simulink model "masterAndSlaveRobots"  (R2021b)
settings: Solver=VariableStepAuto  StartTime=0.0  StopTime=5  RelTol=1e-3
undefined symbols (not defined in the file): A, Bm, Bs, Flp, Km, Ks, Mm, Ms
settings Model: Creator=riccardo  LastModifiedBy=riccardo

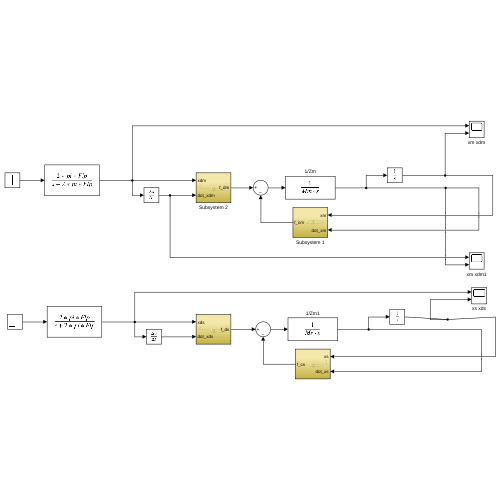
[thumbnail: Simulink's stored preview of the top-level diagram]
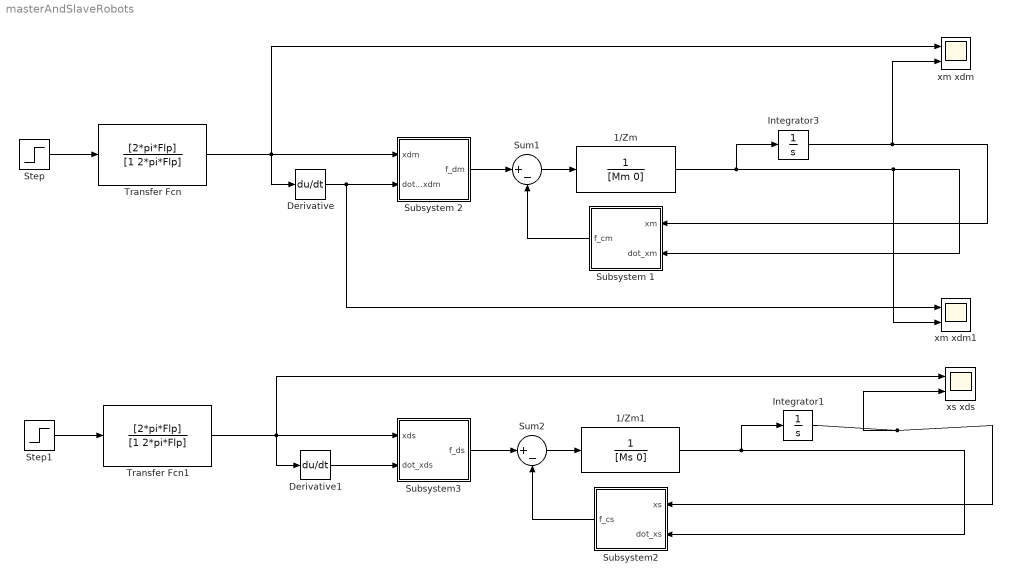
== system masterAndSlaveRobots ==
  1/Zm : TransferFcn  Denominator=[Mm 0]
  1/Zm1 : TransferFcn  Denominator=[Ms 0]
  Derivative : Derivative
  Derivative1 : Derivative
  Integrator1 : Integrator
  Integrator3 : Integrator
  Step : Step  Time=0.5  After=A  SampleTime=0
  Step1 : Step  Time=0.5  After=A  SampleTime=0
  Subsystem 1 : Subsystem
  Subsystem 2 : Subsystem
  Subsystem2 : Subsystem
  Subsystem3 : Subsystem
  Sum1 : Sum  Inputs=|+-
  Sum2 : Sum  Inputs=|+-
  Transfer Fcn : TransferFcn  Numerator=[2*pi*Flp]  Denominator=[1 2*pi*Flp]
  Transfer Fcn1 : TransferFcn  Numerator=[2*pi*Flp]  Denominator=[1 2*pi*Flp]
  xm xdm : Scope  NumInputPorts=2
  xm xdm1 : Scope  NumInputPorts=2
  xs xds : Scope  NumInputPorts=2
  wires:
  Sum1/1 -> 1/Zm/1
  1/Zm/1 -> xm xdm1/2, Subsystem 1/2(dot_xm), Integrator3/1
  Integrator3/1 -> xm xdm/2, Subsystem 1/1(xm)
  Subsystem 1/1(f_cm) -> Sum1/2
  Step/1 -> Transfer Fcn/1
  Transfer Fcn/1 -> xm xdm/1, Derivative/1, Subsystem 2/1(xdm)
  Derivative/1 -> xm xdm1/1, Subsystem 2/2(dot_xdm)
  Subsystem 2/1(f_dm) -> Sum1/1
  Subsystem2/1(f_cs) -> Sum2/2
  Sum2/1 -> 1/Zm1/1
  1/Zm1/1 -> Subsystem2/2(dot_xs), Integrator1/1
  Derivative1/1 -> Subsystem3/2(dot_xds)
  Integrator1/1 -> xs xds/2, Subsystem2/1(xs)
  Step1/1 -> Transfer Fcn1/1
  Subsystem3/1(f_ds) -> Sum2/1
  Transfer Fcn1/1 -> xs xds/1, Derivative1/1, Subsystem3/1(xds)

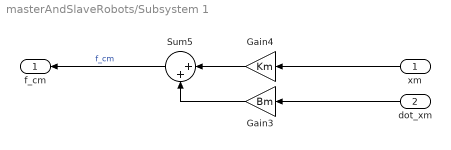
== system masterAndSlaveRobots/Subsystem 1 ==
  xm : Inport
  dot_xm : Inport  Port=2
  Gain3 : Gain  Gain=Bm
  Gain4 : Gain  Gain=Km
  Sum5 : Sum  Inputs=|++
  f_cm : Outport
  wires:
  Gain4/1 -> Sum5/1
  Gain3/1 -> Sum5/2
  dot_xm/1 -> Gain3/1
  Sum5/1 -> f_cm/1  "f_cm"
  xm/1 -> Gain4/1

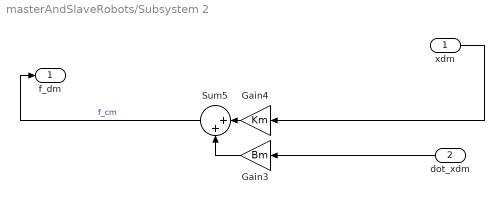
== system masterAndSlaveRobots/Subsystem 2 ==
  xdm : Inport
  dot_xdm : Inport  Port=2
  Gain3 : Gain  Gain=Bm
  Gain4 : Gain  Gain=Km
  Sum5 : Sum  Inputs=|++
  f_dm : Outport
  wires:
  Gain4/1 -> Sum5/1
  Gain3/1 -> Sum5/2
  dot_xdm/1 -> Gain3/1
  Sum5/1 -> f_dm/1  "f_cm"
  xdm/1 -> Gain4/1

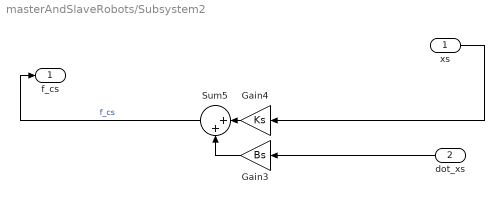
== system masterAndSlaveRobots/Subsystem2 ==
  xs : Inport
  dot_xs : Inport  Port=2
  Gain3 : Gain  Gain=Bs
  Gain4 : Gain  Gain=Ks
  Sum5 : Sum  Inputs=|++
  f_cs : Outport
  wires:
  Gain4/1 -> Sum5/1
  Gain3/1 -> Sum5/2
  dot_xs/1 -> Gain3/1
  Sum5/1 -> f_cs/1  "f_cs"
  xs/1 -> Gain4/1

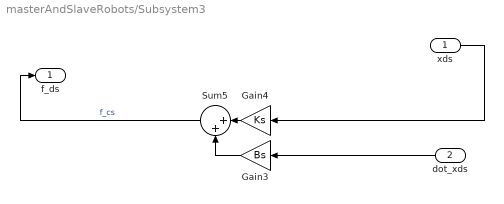
== system masterAndSlaveRobots/Subsystem3 ==
  xds : Inport
  dot_xds : Inport  Port=2
  Gain3 : Gain  Gain=Bs
  Gain4 : Gain  Gain=Ks
  Sum5 : Sum  Inputs=|++
  f_ds : Outport
  wires:
  Gain4/1 -> Sum5/1
  Gain3/1 -> Sum5/2
  dot_xds/1 -> Gain3/1
  Sum5/1 -> f_ds/1  "f_cs"
  xds/1 -> Gain4/1
